simulink model "thyristor_rec"  (R2018a)
settings: Solver=VariableStepAuto  StartTime=0.0  StopTime=100  RelTol=1e-3
libraries: powerlib x12, powerlib_meascontrol x2
settings Model: Creator=ROG  LastModifiedBy=ROG

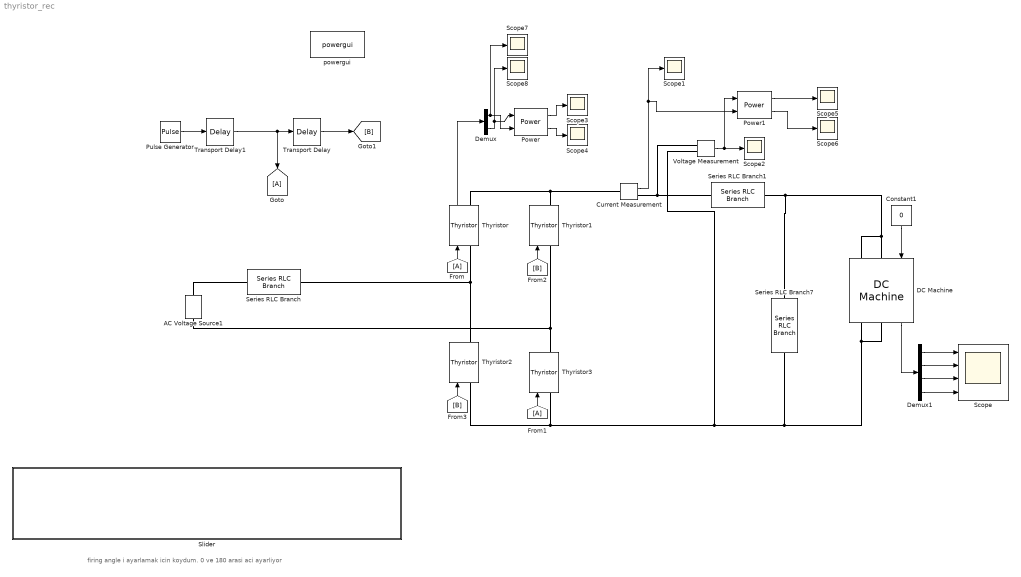
== system thyristor_rec ==
  note: firing angle i ayarlamak icin koydum.
      | 0 ve 180 arasi aci ayarliyor
  AC Voltage Source1 : powerlib/Electrical Sources/AC Voltage Source  Amplitude=325  Phase=0  Frequency=50  SampleTime=0  Measurements=None  BusType=swing  Pref=10e3  Qref=0  Qmin=-inf  Qmax=+inf
  Constant1 : Constant  Value=0
  Current Measurement : powerlib/Measurements/Current Measurement  PhasorSimulation=off  OutputType=Complex  PSBequivalent=0
  DC Machine : powerlib/Machines/DC Machine  PresetModel=No  MechanicalLoad=Torque TL  FieldType=Wound  ShowDetailedParameters=on  MeasurementBus=off  RLa="[ 0.8  0.0125]"  RLf="[ 210  23]"  Laf=1.8  MachineConstant=Torque constant (N.m/A)  Ke=1.8  Kt=1.8  J=4  Bm=0  Tf=0  w0=1  Ifinit=1  TsPowergui=0  TsBlock=-1
  Demux : Demux  Outputs=2
  Demux1 : Demux
  Power : powerlib_meascontrol/Measurements/Power  Freq=60  Vinit=[1, 0]  Iinit=[1, 0]  Ts=0
      settings: SourceProductName=Simscape Power Systems
  Power1 : powerlib_meascontrol/Measurements/Power  Freq=60  Vinit=[1, 0]  Iinit=[1, 0]  Ts=0
      settings: SourceProductName=Simscape Power Systems
  Pulse Generator : DiscretePulseGenerator  PulseType=Time based  Amplitude=5  Period=0.02  PulseWidth=5  PhaseDelay=(0*0.02)/360
  Scope : Scope  NumInputPorts=4
  Scope{1..8} (8 alike) : Scope
  Series RLC Branch : powerlib/Elements/Series RLC Branch  LConnTagsString=__new0  RConnTagsString=__new0  BranchType=L  Resistance=1  Inductance=1e-4  SetiL0=off  InitialCurrent=0  Capacitance=1e-6  Setx0=off  InitialVoltage=0  Measurements=None
  Series RLC Branch1 : powerlib/Elements/Series RLC Branch  LConnTagsString=__new0  RConnTagsString=__new0  BranchType=R  Resistance=10  Inductance=7.2e-3  SetiL0=off  InitialCurrent=0  Capacitance=1e-6  Setx0=off  InitialVoltage=0  Measurements=None
  Series RLC Branch7 : powerlib/Elements/Series RLC Branch  LConnTagsString=__new0  RConnTagsString=__new0  BranchType=C  Resistance=1  Inductance=1e-4  SetiL0=off  InitialCurrent=0  Capacitance=32e-3  Setx0=off  InitialVoltage=0  Measurements=None
  Slider : Subsystem  DialogController=hmiCreateDDGDialog  IsWebBlock=on  mask(MWDashboardBlock){webBlockId=280f5b07-6283-4e31-bf34-1fa9d2077ffd, webBlockType=slider, ShowInLibBrowser=on, ShowInitialText=on, HMISrcModelName=thyristor_rec}
      mask prompts: webBlockId "WebBlock Id"; webBlockType "WebBlock Type"; HMISrcModelName "Source Model"
      mask help: SimulinkHMI:dialogs:SliderDialogDesc
      mask Help: helpview([docroot '/mapfiles/simulink.map'], 'hmi_slider')
      mask Display:
      | if strcmp(get_param(bdroot(gcb),'BlockDiagramType'), 'library')
      |     image([(matlabroot) '/toolbox/simulink/hmi/icons/Slider.png']);
      | end
  Thyristor{,1..3} (4 alike) : powerlib/Power Electronics/Thyristor  Ron=0.001  Lon=0  Vf=0.8  IC=0  Rs=500  Cs=250e-9  Measurements=on
  Transport Delay : TransportDelay  DelayTime=0.01
  Transport Delay1 : TransportDelay  DelayTime=0
  Voltage Measurement : powerlib/Measurements/Voltage Measurement  PhasorSimulation=off  OutputType=Complex  PSBequivalent=0
  powergui : powerlib/powergui  Priority=1  SimulationMode=Discrete  SampleTime=50e-6  frequency=60  Iterations=50  frequencyindice=0  Pbase=100e6  ErrMax=1e-4  UnitsV=kV  UnitsW=MW  buscounter=0  FunctionMessages=off  echomessages=off  EnableUseOfTLC=off  CurrentSourceSwitches=off  DisableSnubberDevices=off  DisableRonSwitches=off  DisableVfSwitches=off  DisplayEquations=off  SolverType=Tustin/Backward Euler (TBE)  Interpol=off  ExternalGateDelay=off  methode=off  Ts=100  x0status=blocks  SPID=off  SwTol=0  HookPort=off  RestoreLinks=warning  ResistiveCurrentMeasurement=off  Frange=[0:2:500]  Ylog=off  Xlog=on  ShowGrid=off  save=off  variable=ZData  structure=0  ZoomFFT=off  StartTime=0.0  cycles=1  DisplayStyle=1  fundamental=60  FreqAxis=off  MaxFrequency=1000  frequencyindicesteady=1  RmsSteady=1  display=off
  wires:
  Constant1/1 -> DC Machine/1
  DC Machine/1 -> Demux1/1
  Demux1/1 -> Scope/1
  Demux1/2 -> Scope/2
  Demux1/3 -> Scope/3
  Demux1/4 -> Scope/4
  Current Measurement/1 -> Power1/2, Scope1/1
  Voltage Measurement/1 -> Power1/1, Scope2/1
  Thyristor/1 -> Demux/1
  Power/1 -> Scope3/1
  Power/2 -> Scope4/1
  Power1/1 -> Scope5/1
  Power1/2 -> Scope6/1
  Demux/1 -> Scope7/1, Power/2
  Demux/2 -> Scope8/1, Power/1
  [A] -> Thyristor/1
  [B] -> Thyristor2/1
  Transport Delay/1 -> [B]
  [B] -> Thyristor1/1
  [A] -> Thyristor3/1
  Transport Delay1/1 -> [A], Transport Delay/1
  Pulse Generator/1 -> Transport Delay1/1
  connections:
  Thyristor3/RConn1 -- AC Voltage Source1/LConn1 -- Thyristor1/LConn1
  Thyristor/RConn1 -- Current Measurement/LConn1 -- Thyristor1/RConn1
  Series RLC Branch/LConn1 -- AC Voltage Source1/RConn1
  Series RLC Branch1/LConn1 -- Current Measurement/RConn1 -- Voltage Measurement/LConn1
  Thyristor2/LConn1 -- DC Machine/RConn1 -- DC Machine/RConn2 -- Series RLC Branch7/RConn1 -- Voltage Measurement/LConn2 -- Thyristor3/LConn1
  Thyristor/LConn1 -- Thyristor2/RConn1 -- Series RLC Branch/RConn1
  Series RLC Branch7/LConn1 -- Series RLC Branch1/RConn1 -- DC Machine/LConn2 -- DC Machine/LConn1

== system thyristor_rec/Slider ==
